simulink model "clk_tree_1"  (Simulink 7.0)
settings: Solver=ode45  StartTime=0.0  StopTime=40e-6  MaxStep=0.1e-9  RelTol=1e-3
InitFcn:
  | bit_rate=400e6;
libraries: powerlib x35, simulink x2, commrandsrc2 x1, dspbuff3 x1, dspsnks4 x1
settings Model: Creator=dbenson  LastModifiedBy=dbenson
settings OptimizationCC: InlineInvariantSignals=on
settings DebuggingCC: SaveWithParameterizedLinksMsg=none  SignalResolutionControl=TryResolveAllWithWarning  MultiTaskDSMMsg=warning  MultiTaskCondExecSysMsg=none  StrictBusMsg=None
settings RTWCC: IncludeERTFirstTime=on
settings GRTTargetCC: TargetFcnLib=ansi_tfl_tmw.mat

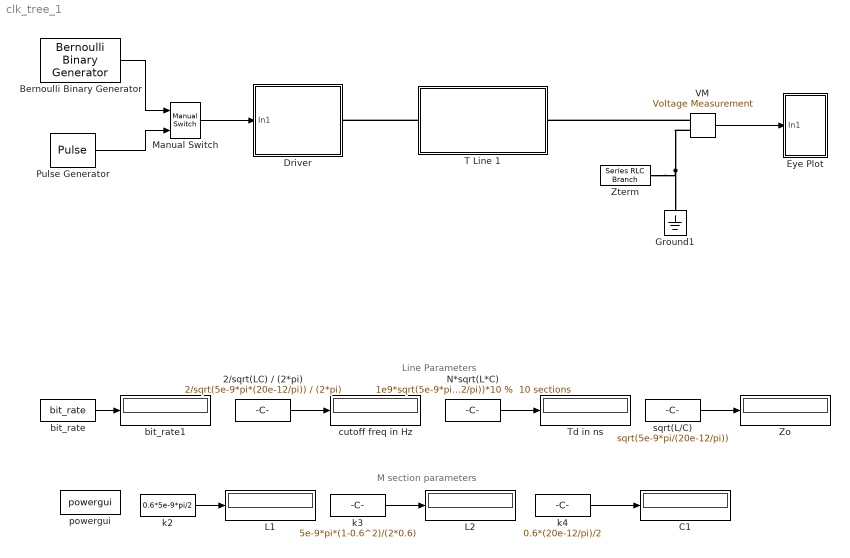
== system clk_tree_1 ==
  note: Line Parameters
  note: M section parameters
  2/sqrt(LC) / (2*pi) : Constant  Value=2/sqrt(5e-9*pi*(20e-12/pi)) / (2*pi)  OutDataType=sfix(16)  OutScaling=2^0
  Bernoulli Binary Generator : commrandsrc2/Bernoulli Binary Generator  DialogController=commDDGCreate  DialogControllerArgs=DataTag0  SystemSampleTime=-1  P=0.5  seed=61  Ts=1/bit_rate  frameBased=off  sampPerFrame=1  orient=off  outDataType=double
  C1 : Display
  Driver : Subsystem
  Eye Plot : Subsystem
  Ground1 : powerlib/Elements/Ground  Orientation=down  DialogController=POWERSYS.PowerSysDialog  PhysicalDomain=powersysdomain  SubClassName=unknown  LeftPortType=p1  RightPortType=p1  LConnTagsString=a
  L1 : Display
  L2 : Display
  Manual Switch : simulink/Signal Routing/Manual Switch  SystemSampleTime=-1  sw=1  action=0  varsize=off
  N*sqrt(L*C) : Constant  Value="1e9*sqrt(5e-9*pi*(20e-12/pi))*10 %  10 sections"  OutDataType=sfix(16)  OutScaling=2^0
  Pulse Generator : DiscretePulseGenerator  PulseType=Time based  Period=2/bit_rate  PulseWidth=50
  T Line 1 : Subsystem
  Td in ns : Display
  VM : powerlib/Measurements/Voltage Measurement  DialogController=POWERSYS.PowerSysDialog  SystemSampleTime=-1  PhasorSimulation=off  OutputType=Complex  PSBequivalent=0
  Zo : Display
  Zterm : powerlib/Elements/Series RLC Branch  DialogController=POWERSYS.PowerSysDialog  PhysicalDomain=powersysdomain  SubClassName=unknown  LeftPortType=p1  RightPortType=p1  LConnTagsString=__new0  RConnTagsString=__new0  BranchType=R  Resistance=50  Inductance=1e-3  SetiL0=off  InitialCurrent=0  Capacitance=1e-6  Setx0=off  InitialVoltage=0  Measurements=None
  bit_rate : Constant  Value=bit_rate  OutDataType=sfix(16)  OutScaling=2^0
  bit_rate1 : Display
  cutoff freq in Hz : Display
  k2 : Constant  Value=0.6*5e-9*pi/2  OutDataType=sfix(16)  OutScaling=2^0
  k3 : Constant  Value=5e-9*pi*(1-0.6^2)/(2*0.6)  OutDataType=sfix(16)  OutScaling=2^0
  k4 : Constant  Value=0.6*(20e-12/pi)/2  OutDataType=sfix(16)  OutScaling=2^0
  powergui : powerlib/powergui  SystemSampleTime=-1  SimulationMode=Continuous  SampleTime=50e-6  echomessages=off  RestoreLinks=warning  x0status=blocks  Frange=[0:2:500]  Ylog=off  Xlog=on  ShowGrid=off  save=off  variable=ZData  ZoomFFT=on  StartTime=0.0  cycles=1  DisplayStyle=1  fundamental=60  FreqAxis=off  MaxFrequency=1000  frequencyindice=0  frequencyindicesteady=1  RmsSteady=1  display=off  Ts=0  frequency=60  methode=off  HookPort=off  Interpol=off  SPID=off  FunctionMessages=off
  sqrt(L/C) : Constant  Value=sqrt(5e-9*pi/(20e-12/pi))  OutDataType=sfix(16)  OutScaling=2^0
  wires:
  sqrt(L/C)/1 -> Zo/1
  N*sqrt(L*C)/1 -> Td in ns/1
  k2/1 -> L1/1
  k3/1 -> L2/1
  k4/1 -> C1/1
  2/sqrt(LC) / (2*pi)/1 -> cutoff freq in Hz/1
  VM/1 -> Eye Plot/1(In1)
  bit_rate/1 -> bit_rate1/1
  Pulse Generator/1 -> Manual Switch/2
  Bernoulli Binary Generator/1 -> Manual Switch/1
  Manual Switch/1 -> Driver/1(In1)
  connections:
  T Line 1/LConn1 -- Driver/RConn1
  VM/LConn2 -- Ground1/LConn1 -- Zterm/RConn1
  VM/LConn1 -- T Line 1/RConn1

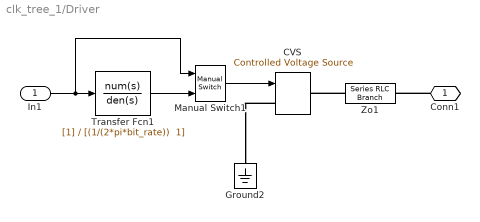
== system clk_tree_1/Driver ==
  In1 : Inport
  CVS : powerlib/Electrical Sources/Controlled Voltage Source  Description=source block  DialogController=POWERSYS.PowerSysDialog  SystemSampleTime=-1  Initialize=off  Source_Type=AC  Amplitude=0  Phase=0  Frequency=0  Measurements=None
      settings: AttributesFormatString=\n
  Ground2 : powerlib/Elements/Ground  Orientation=down  DialogController=POWERSYS.PowerSysDialog  PhysicalDomain=powersysdomain  SubClassName=unknown  LeftPortType=p1  RightPortType=p1  LConnTagsString=a
  Manual Switch1 : simulink/Signal Routing/Manual Switch  SystemSampleTime=-1  sw=0  action=0  varsize=off
  Transfer Fcn1 : TransferFcn  Denominator="[(1/(2*pi*bit_rate))  1]"
  Zo1 : powerlib/Elements/Series RLC Branch  DialogController=POWERSYS.PowerSysDialog  PhysicalDomain=powersysdomain  SubClassName=unknown  LeftPortType=p1  RightPortType=p1  LConnTagsString=__new0  RConnTagsString=__new0  BranchType=R  Resistance=50  Inductance=1e-3  SetiL0=off  InitialCurrent=0  Capacitance=1e-6  Setx0=off  InitialVoltage=0  Measurements=None
  Conn1 : PMIOPort  Orientation=left  Port=1  Side=Right
  wires:
  In1/1 -> Manual Switch1/1, Transfer Fcn1/1
  Manual Switch1/1 -> CVS/1
  Transfer Fcn1/1 -> Manual Switch1/2
  connections:
  CVS/LConn1 -- Ground2/LConn1
  Zo1/LConn1 -- CVS/RConn1
  Conn1/RConn1 -- Zo1/RConn1

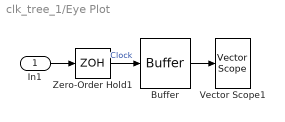
== system clk_tree_1/Eye Plot ==
  In1 : Inport
  Buffer : dspbuff3/Buffer  N=200  V=0  ic=0
  Vector Scope1 : dspsnks4/Vector Scope  DialogController=dspdialog.VectorScope  DialogControllerArgs=DataTag1  ScopeProperties=on  Domain=User-defined  HorizSpan=1  DisplayProperties=off  AxisGrid=on  Memory=on  FrameNumber=on  AxisLegend=off  AxisZoom=off  OpenScopeAtSimStart=on  OpenScopeImmediately=off  FigPos=[3 39 417 270]  AxisProperties=off  XUnits=Hertz  XRange=[0...Fs/2]  InheritXIncr=off  XIncr=.01/bit_rate  XLabel=Time  XLimit=Auto  XMin=0  XMax=1  XStart=0  YUnits=dB  YLabel=Amplitude  LineProperties=off  LineColors=[0 0 1]|[1 0 0]
      settings: YMin=-0.298875449569035  YMax=1.30250670189524
  Zero-Order Hold1 : ZeroOrderHold  SampleTime=.01/bit_rate
  wires:
  Zero-Order Hold1/1 -> Buffer/1  "Clock"
  Buffer/1 -> Vector Scope1/1
  In1/1 -> Zero-Order Hold1/1

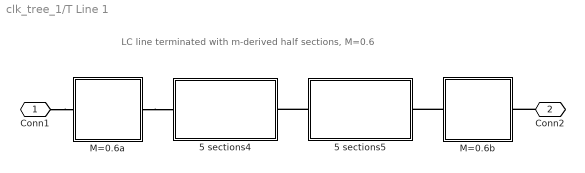
== system clk_tree_1/T Line 1 ==
  note: LC line terminated with m-derived half sections, M=0.6
  5 sections4 : Subsystem
  5 sections5 : Subsystem
  M=0.6a : Subsystem
  M=0.6b : Subsystem
  Conn1 : PMIOPort  Port=1  Side=Left
  Conn2 : PMIOPort  Orientation=left  Port=2  Side=Right
  connections:
  M=0.6a/RConn1 -- 5 sections4/LConn1
  5 sections5/LConn1 -- 5 sections4/RConn1
  M=0.6b/LConn1 -- 5 sections5/RConn1
  Conn1/RConn1 -- M=0.6a/LConn1
  Conn2/RConn1 -- M=0.6b/RConn1

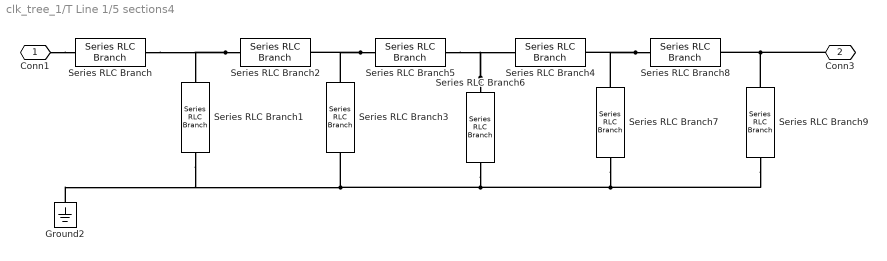
== system clk_tree_1/T Line 1/5 sections4 ==
  Ground2 : powerlib/Elements/Ground  Orientation=down  DialogController=POWERSYS.PowerSysDialog  PhysicalDomain=powersysdomain  SubClassName=unknown  LeftPortType=p1  RightPortType=p1  LConnTagsString=a
  Series RLC Branch{,2,4..5,8} (5 alike) : powerlib/Elements/Series RLC Branch  DialogController=POWERSYS.PowerSysDialog  PhysicalDomain=powersysdomain  SubClassName=unknown  LeftPortType=p1  RightPortType=p1  LConnTagsString=__new0  RConnTagsString=__new0  BranchType=L  Resistance=1.0  Inductance=5*pi*1e-9  SetiL0=off  InitialCurrent=0  Capacitance=1.0  Setx0=off  InitialVoltage=0  Measurements=None
  Series RLC Branch{1,3,6..7,9} (5 alike) : powerlib/Elements/Series RLC Branch  Orientation=down  DialogController=POWERSYS.PowerSysDialog  PhysicalDomain=powersysdomain  SubClassName=unknown  LeftPortType=p1  RightPortType=p1  LConnTagsString=__new0  RConnTagsString=__new0  BranchType=C  Resistance=1.0  Inductance=1.0  SetiL0=off  InitialCurrent=0  Capacitance=20e-12/pi  Setx0=off  InitialVoltage=0  Measurements=None
  Conn1 : PMIOPort  Port=1  Side=Left
  Conn3 : PMIOPort  Orientation=left  Port=2  Side=Right
  connections:
  Conn1/RConn1 -- Series RLC Branch/LConn1
  Conn3/RConn1 -- Series RLC Branch8/RConn1 -- Series RLC Branch9/LConn1
  Series RLC Branch8/LConn1 -- Series RLC Branch4/RConn1 -- Series RLC Branch7/LConn1
  Series RLC Branch6/LConn1 -- Series RLC Branch4/LConn1 -- Series RLC Branch5/RConn1
  Series RLC Branch5/LConn1 -- Series RLC Branch2/RConn1 -- Series RLC Branch3/LConn1
  Series RLC Branch9/RConn1 -- Series RLC Branch7/RConn1 -- Series RLC Branch1/RConn1 -- Ground2/LConn1 -- Series RLC Branch3/RConn1 -- Series RLC Branch6/RConn1
  Series RLC Branch2/LConn1 -- Series RLC Branch1/LConn1 -- Series RLC Branch/RConn1

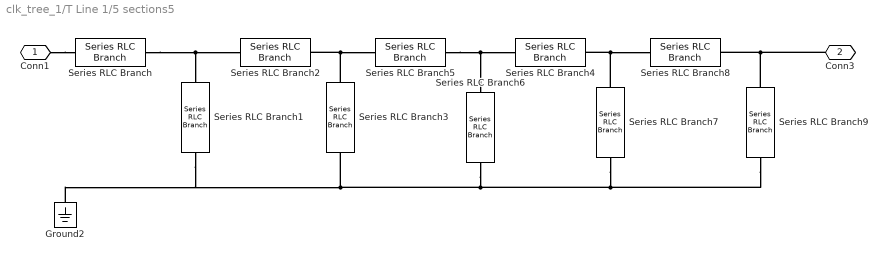
== system clk_tree_1/T Line 1/5 sections5 ==
  Ground2 : powerlib/Elements/Ground  Orientation=down  DialogController=POWERSYS.PowerSysDialog  PhysicalDomain=powersysdomain  SubClassName=unknown  LeftPortType=p1  RightPortType=p1  LConnTagsString=a
  Series RLC Branch{,2,4..5,8} (5 alike) : powerlib/Elements/Series RLC Branch  DialogController=POWERSYS.PowerSysDialog  PhysicalDomain=powersysdomain  SubClassName=unknown  LeftPortType=p1  RightPortType=p1  LConnTagsString=__new0  RConnTagsString=__new0  BranchType=L  Resistance=1.0  Inductance=5*pi*1e-9  SetiL0=off  InitialCurrent=0  Capacitance=1.0  Setx0=off  InitialVoltage=0  Measurements=None
  Series RLC Branch{1,3,6..7,9} (5 alike) : powerlib/Elements/Series RLC Branch  Orientation=down  DialogController=POWERSYS.PowerSysDialog  PhysicalDomain=powersysdomain  SubClassName=unknown  LeftPortType=p1  RightPortType=p1  LConnTagsString=__new0  RConnTagsString=__new0  BranchType=C  Resistance=1.0  Inductance=1.0  SetiL0=off  InitialCurrent=0  Capacitance=20e-12/pi  Setx0=off  InitialVoltage=0  Measurements=None
  Conn1 : PMIOPort  Port=1  Side=Left
  Conn3 : PMIOPort  Orientation=left  Port=2  Side=Right
  connections:
  Series RLC Branch/RConn1 -- Series RLC Branch1/LConn1 -- Series RLC Branch2/LConn1
  Series RLC Branch9/RConn1 -- Series RLC Branch6/RConn1 -- Series RLC Branch3/RConn1 -- Series RLC Branch1/RConn1 -- Ground2/LConn1 -- Series RLC Branch7/RConn1
  Series RLC Branch3/LConn1 -- Series RLC Branch2/RConn1 -- Series RLC Branch5/LConn1
  Series RLC Branch5/RConn1 -- Series RLC Branch4/LConn1 -- Series RLC Branch6/LConn1
  Series RLC Branch7/LConn1 -- Series RLC Branch4/RConn1 -- Series RLC Branch8/LConn1
  Series RLC Branch9/LConn1 -- Series RLC Branch8/RConn1 -- Conn3/RConn1
  Conn1/RConn1 -- Series RLC Branch/LConn1

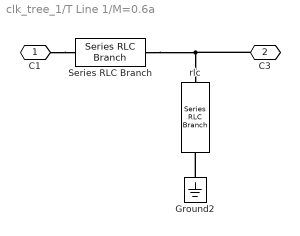
== system clk_tree_1/T Line 1/M=0.6a ==
  Ground2 : powerlib/Elements/Ground  Orientation=down  DialogController=POWERSYS.PowerSysDialog  PhysicalDomain=powersysdomain  SubClassName=unknown  LeftPortType=p1  RightPortType=p1  LConnTagsString=a
  Series RLC Branch : powerlib/Elements/Series RLC Branch  DialogController=POWERSYS.PowerSysDialog  PhysicalDomain=powersysdomain  SubClassName=unknown  LeftPortType=p1  RightPortType=p1  LConnTagsString=__new0  RConnTagsString=__new0  BranchType=L  Resistance=1.0  Inductance=4.712e-9  SetiL0=off  InitialCurrent=0  Capacitance=1.0  Setx0=off  InitialVoltage=0  Measurements=None
  rlc : powerlib/Elements/Series RLC Branch  Orientation=down  DialogController=POWERSYS.PowerSysDialog  PhysicalDomain=powersysdomain  SubClassName=unknown  LeftPortType=p1  RightPortType=p1  LConnTagsString=__new0  RConnTagsString=__new0  BranchType=LC  Resistance=1.0  Inductance=8.378e-9  SetiL0=off  InitialCurrent=0  Capacitance=1.91e-12  Setx0=off  InitialVoltage=0  Measurements=None
  C1 : PMIOPort  Port=1  Side=Left
  C3 : PMIOPort  Orientation=left  Port=2  Side=Right
  connections:
  C3/RConn1 -- rlc/LConn1 -- Series RLC Branch/RConn1
  C1/RConn1 -- Series RLC Branch/LConn1
  Ground2/LConn1 -- rlc/RConn1

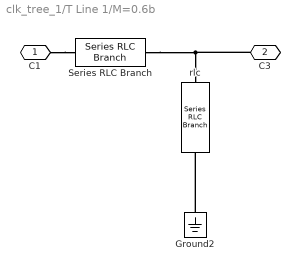
== system clk_tree_1/T Line 1/M=0.6b ==
  Ground2 : powerlib/Elements/Ground  Orientation=down  DialogController=POWERSYS.PowerSysDialog  PhysicalDomain=powersysdomain  SubClassName=unknown  LeftPortType=p1  RightPortType=p1  LConnTagsString=a
  Series RLC Branch : powerlib/Elements/Series RLC Branch  DialogController=POWERSYS.PowerSysDialog  PhysicalDomain=powersysdomain  SubClassName=unknown  LeftPortType=p1  RightPortType=p1  LConnTagsString=__new0  RConnTagsString=__new0  BranchType=L  Resistance=1.0  Inductance=4.712e-9  SetiL0=off  InitialCurrent=0  Capacitance=1.0  Setx0=off  InitialVoltage=0  Measurements=None
  rlc : powerlib/Elements/Series RLC Branch  Orientation=down  DialogController=POWERSYS.PowerSysDialog  PhysicalDomain=powersysdomain  SubClassName=unknown  LeftPortType=p1  RightPortType=p1  LConnTagsString=__new0  RConnTagsString=__new0  BranchType=LC  Resistance=1.0  Inductance=8.378e-9  SetiL0=off  InitialCurrent=0  Capacitance=1.91e-12  Setx0=off  InitialVoltage=0  Measurements=None
  C1 : PMIOPort  Port=1  Side=Left
  C3 : PMIOPort  Orientation=left  Port=2  Side=Right
  connections:
  C1/RConn1 -- Series RLC Branch/LConn1
  Ground2/LConn1 -- rlc/RConn1
  Series RLC Branch/RConn1 -- rlc/LConn1 -- C3/RConn1
